simulink model "gm_SS_debug"  (R2025b)
settings: Solver=VariableStepAuto  StartTime=0.0  StopTime=10.0  RelTol=1e-3
settings Model: Creator=info  LastModifiedBy=info
settings OptimizationCC: BlockReduction=off  ConditionallyExecuteInputs=off  DefaultParameterBehavior=Inlined
settings DebuggingCC: AlgebraicLoopMsg=error  InheritedTsInSrcMsg=none
settings HardwareCC: ProdBitPerPointer=32.0  ProdBitPerSizeT=32.0  ProdBitPerPtrDiffT=32.0  ProdLargestAtomicFloat=None  ProdIntDivRoundTo=Undefined  ProdEndianess=Unspecified  ProdWordSize=32.0  ProdHWDeviceType=ASIC/FPGA->ASIC/FPGA  TargetBitPerPointer=64.0  TargetBitPerSizeT=64.0  TargetBitPerPtrDiffT=64.0  TargetLongLongMode=on  TargetIntDivRoundTo=Zero  TargetEndianess=LittleEndian  TargetWordSize=64.0  TargetHWDeviceType=Custom Processor->MATLAB Host Computer  ProdEqTarget=off

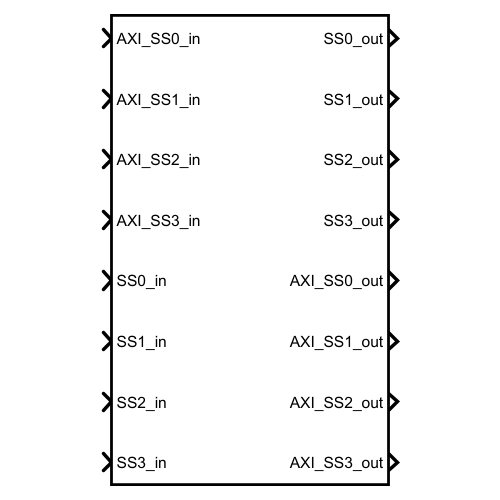
[thumbnail: Simulink's stored preview of the top-level diagram]
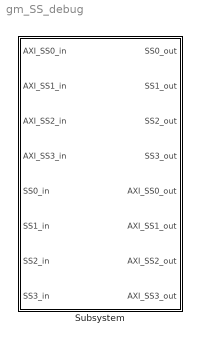
== system gm_SS_debug ==
  Subsystem : Subsystem  TreatAsAtomicUnit=on

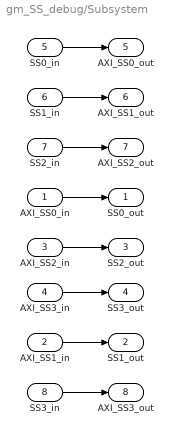
== system gm_SS_debug/Subsystem ==
  AXI_SS0_in : Inport  OutDataTypeStr=boolean  PortDimensions=1
  AXI_SS1_in : Inport  Port=2  OutDataTypeStr=boolean  PortDimensions=1
  AXI_SS2_in : Inport  Port=3  OutDataTypeStr=boolean  PortDimensions=1
  AXI_SS3_in : Inport  Port=4  OutDataTypeStr=boolean  PortDimensions=1
  SS0_in : Inport  Port=5  OutDataTypeStr=boolean  PortDimensions=1
  SS1_in : Inport  Port=6  OutDataTypeStr=boolean  PortDimensions=1
  SS2_in : Inport  Port=7  OutDataTypeStr=boolean  PortDimensions=1
  SS3_in : Inport  Port=8  OutDataTypeStr=boolean  PortDimensions=1
  SS0_out : Outport  OutDataTypeStr=boolean
  SS1_out : Outport  Port=2  OutDataTypeStr=boolean
  SS2_out : Outport  Port=3  OutDataTypeStr=boolean
  SS3_out : Outport  Port=4  OutDataTypeStr=boolean
  AXI_SS0_out : Outport  Port=5  OutDataTypeStr=boolean
  AXI_SS1_out : Outport  Port=6  OutDataTypeStr=boolean
  AXI_SS2_out : Outport  Port=7  OutDataTypeStr=boolean
  AXI_SS3_out : Outport  Port=8  OutDataTypeStr=boolean
  wires:
  AXI_SS1_in/1 -> SS1_out/1
  AXI_SS3_in/1 -> SS3_out/1
  SS1_in/1 -> AXI_SS1_out/1
  SS0_in/1 -> AXI_SS0_out/1
  SS3_in/1 -> AXI_SS3_out/1
  AXI_SS0_in/1 -> SS0_out/1
  SS2_in/1 -> AXI_SS2_out/1
  AXI_SS2_in/1 -> SS2_out/1
